simulink model "SimV6"  (R2024b)
settings: Solver=FixedStepAuto  StartTime=0.0  StopTime=5  RelTol=1e-3
model workspace (MAT data in the model file):
  Sig = Simulink.Signal
  Sig.Dimensions = -1
  Sig.DimensionsMode = 'auto'
  Sig.Complexity = 'auto'
  Sig.SampleTime = -1
  Sig.SamplingMode = 'auto'
  Sig.DataType = 'auto'
values from neighbouring files (symbols this model uses):
  CanaryCarrierFrequency = 20000.0    [ConfigData.sldd]
  CanaryDataRate = 100.0    [ConfigData.sldd]
  DataAmplitude = 10.0    [ConfigData.sldd]
  FmDecoderFrameSize = 128.0    [ConfigData.sldd]
  FmFrequencyDifferential = 400.0    [ConfigData.sldd]
  PreConvolveDownsample = 32.0    [ConfigData.sldd]
  SampleRate = 48000.0    [ConfigData.sldd]
  WalshCodeCache = 1.0 1.0 1.0 1.0 1.0 1.0 1.0 1.0 1.0 1.0 1.0 1.0 1.0 1.0 1.0 1.0 1.0 1.0 1.0 1.0 1.0 1.0 1.0 1.0 1.0 1.0 1.0 1.0 1.0 1.0 1.0 1.0 1.0 1.0 1.0 1.0 1.0 1.0 1.0 1.0 1.0 1.0 1.0 1.0 1.0 1.0 1.0 1.0 1.0 1.0 1.0 1.0 1.0 1.0 -1.0 -1.0 -1.0 -1.0 -1.0 -1.0 -1.0 -1.0 -1.0 -1.0 -1.0 -1.0 -1.0 -1.0 -1.0 -1.0 -1.0 -1.0 -1.0 -1.0 -1.0 -1.0 -1.0 -1.0 -1.0 -1.0 -1.0 -1.0 -1.0 -1.0 -1.0 -1.0 -1.0 -1.0 -1.0 -1.0 -1.0    [ConfigData.sldd]
  WalshCodeIndex = 3.0 9.0    [ConfigData.sldd]
libraries: dspstat3 x3, dspfdesign x3, audiosources x2, eeGeneralControl x2, commseqgen3 x2, commchan3 x1, dspsnks4 x1, simulink x1, dspsrcs4 x1, dspsigops x1
settings Model: DataDictionary=ConfigData.sldd  SimulationMode=accelerator  PauseTimes=4.5  PacingRate=0.007100  Creator=calum  LastModifiedBy=calum
settings SolverCC: AllowMultiTaskInputOutput=on  ConcurrentTasks=on  AutoInsertRateTranBlk=on
settings OptimizationCC: StateBitsets=on  DataBitsets=on  SimCompilerOptimization=on  AccelVerboseBuild=on  MultiThreadedLoops=on
settings DebuggingCC: IntegerOverflowMsg=none  IntegerSaturationMsg=none
settings HardwareCC: ProdBitPerLong=64  ProdLongLongMode=on  ProdHWDeviceType=Intel->x86-64 (Linux 64)
settings ModelReferenceCC: UpdateModelReferenceTargets=IfOutOfDate  EnableParallelModelReferenceBuilds=on  ParallelModelReferenceMATLABWorkerInit=Copy Base Workspace
settings SFSimCC: SimCtrlC=off  SimHardwareAcceleration=native
settings RTWCC: Description=Simulink Desktop Real-Time (ERT)  SystemTargetFile=sldrtert.tlc  TemplateMakefile=sldrtert.tmf  GenerateReport=on  Toolchain=GNU gcc/g++ | gmake (64-bit Linux)  BuildConfiguration=Specify  LaunchReport=on  TargetLang=C++  RTWCompilerOptimization=on  CheckMdlBeforeBuild=Warning
settings CodeAppCC: MaxIdLength=95  MATLABSourceComments=on
settings SimulinkDesktopRealTimeERTCC: TargetFcnLib=ansi_tfl_table_tmw.mat  TargetLibSuffix=_sldrt.a  TargetPreCompLibLocation=/home/calum/.local/matlab/2024b/toolbox/sldrt/lib/glnxa64  GenFloatMathFcnCalls=NOT IN USE  TargetLangStandard=C++11 (ISO)  CodeReplacementLibrary=None  UtilityFuncGeneration=Auto  MultiwordTypeDef=System defined  MultiwordLength=2048  DynamicStringBufferSize=256  GenerateFullHeader=on  InferredTypesCompatibility=off  GenerateSampleERTMain=off  GenerateTestInterfaces=off  ModelReferenceCompliant=on  ParMdlRefBuildCompliant=on  CompOptLevelCompliant=on  ConcurrentExecutionCompliant=off  IncludeMdlTerminateFcn=on  CombineOutputUpdateFcns=off  CombineSignalStateStructs=off  GroupInternalDataByFunction=off  SuppressErrorStatus=off  IncludeFileDelimiter=Auto  ERTCustomFileBanners=off  SupportAbsoluteTime=on  LogVarNameModifier=rt_  MatFileLogging=off  CodeInterfacePackaging=Nonreusable function  PurelyIntegerCode=off  SupportNonFinite=on  SupportComplex=on  SupportContinuousTime=on  SupportNonInlinedSFcns=on  RemoveDisableFunc=off  RemoveResetFunc=off  SupportVariableSizeSignals=on  ParenthesesLevel=Nominal  CastingMode=Nominal  MATLABClassNameForMDSCustomization=Simulink.SoftwareTarget.TargetSpecificTriggerConfigurationBase  ModelStepFunctionPrototypeControlCompliant=off  CPPClassGenCompliant=off  AutosarCompliant=off  MDXCompliant=off  GRTInterface=off  GenerateAllocFcn=off  UseToolchainInfoCompliant=off  GenerateSharedConstants=on  CoderGroups=[]  AccessMethods=[]  LookupTableObjectStructAxisOrder=1,2,3,4,...  LUTObjectStructOrderExplicitValues=Size,Breakpoints,Table  LUTObjectStructOrderEvenSpacing=Size,Breakpoints,Table  ArrayLayout=Column-major  UnsupportedSFcnMsg=error  ERTHeaderFileRootName=$R$E  ERTSourceFileRootName=$R$E  ERTDataFileRootName=$R_data  InstructionSetFMA=on  OptimizeReductions=on  LogToMDFFile=off  GenerateASAP2=off  DSAsUniqueAccess=off  ExtMode=on  ExtModeTransport=0  ExtModeStaticAlloc=off  ExtModeAutomaticAllocSize=on  ExtModeMaxTrigDuration=10  ExtModeStaticAllocSize=1000000  ExtModeTesting=off  ExtModeMexFile=sldrtext  ExtModeIntrfLevel=Level1  InlinedParameterPlacement=Hierarchical  TargetOS=BareBoardExample  MultiInstanceErrorCode=Error  RootIOFormat=Individual arguments  RTWCAPISignals=off  RTWCAPIParams=off  RTWCAPIStates=off  RTWCAPIRootIO=off  ERTSrcFileBannerTemplate=ert_code_template.cgt  ERTHdrFileBannerTemplate=ert_code_template.cgt  ERTDataSrcFileTemplate=ert_code_template.cgt  ERTDataHdrFileTemplate=ert_code_template.cgt  ERTCustomFileTemplate=example_file_process.tlc  EnableDataOwnership=off  SignalDisplayLevel=10  ParamTuneLevel=10  GlobalDataDefinition=Auto  DataDefinitionFile=global.c  GlobalDataReference=Auto  ERTFilePackagingFormat=Modular  RateTransitionBlockCode=Inline  DataReferenceFile=global.h  PreserveExpressionOrder=off  PreserveIfCondition=off  ConvertIfToSwitch=off  PreserveExternInFcnDecls=on  PreserveStaticInFcnDecls=on  SuppressUnreachableDefaultCases=off  EnableSignedLeftShifts=on  EnableSignedRightShifts=on  ImplementImageWithCVMat=off  IndentStyle=K&R  IndentSize=2  NewlineStyle=Default  MaxLineWidth=80  EnableUserReplacementTypes=off  MaxIdInt64=MAX_int64_T  MinIdInt64=MIN_int64_T  MaxIdUint64=MAX_uint64_T  MaxIdInt32=MAX_int32_T  MinIdInt32=MIN_int32_T  MaxIdUint32=MAX_uint32_T  MaxIdInt16=MAX_int16_T  MinIdInt16=MIN_int16_T  MaxIdUint16=MAX_uint16_T  MaxIdInt8=MAX_int8_T  MinIdInt8=MIN_int8_T  MaxIdUint8=MAX_uint8_T  BooleanTrueId=true  BooleanFalseId=false  MemSecPackage=--- None ---  MemSecDataConstants=Default  MemSecDataIO=Default  MemSecDataInternal=Default  MemSecDataParameters=Default  MemSecFuncInitTerm=Default  MemSecFuncExecute=Default  MemSecFuncSharedUtil=Default  GroupConstants=Default  GroupRootInputs=Default  GroupRootOutputs=Default  GroupInternal=Default  GroupParameters=Default  GroupDataTransfer=Default  GroupSharedLocalDataStores=Default  GroupInstanceSpecificParameters=Default  GroupModelData=Default  ArrayContainerType=C-style array  DynamicArrayContainerType=std::vector  CCListing=off  RebuildAll=off

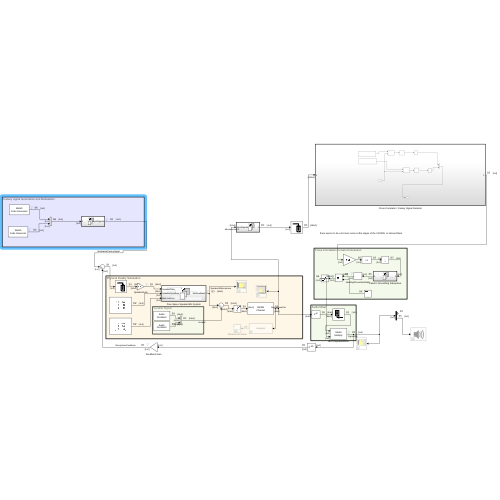
[thumbnail: Simulink's stored preview of the top-level diagram]
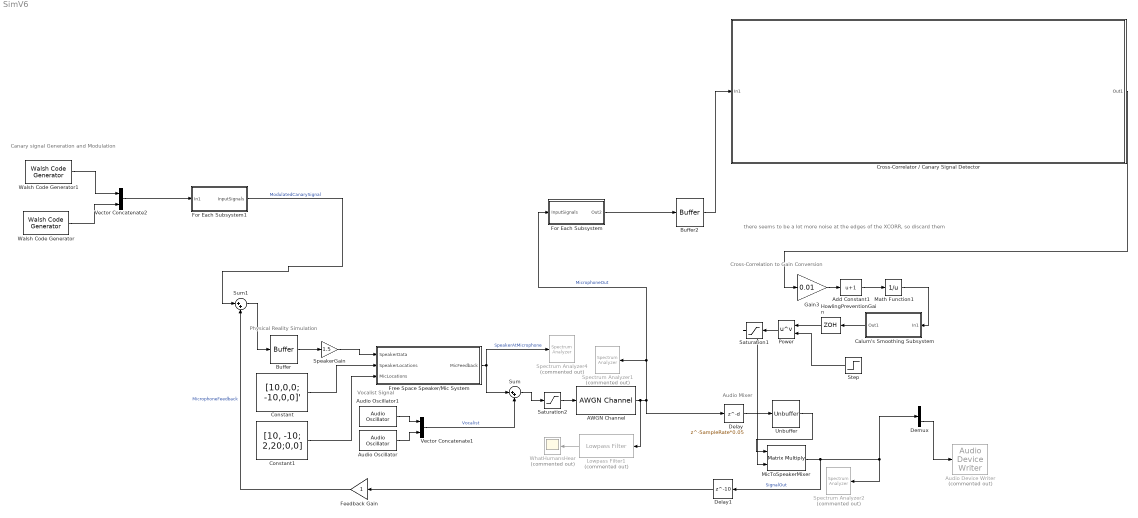
== system SimV6 ==
  note: Canary signal Generation and Modulation
  note: Audio Mixer
  note: Physical Reality Simulation
  note: Vocalist Signal
  note: Cross-Correlation to Gain Conversion
  note: there seems to be a lot more noise at the edges of the XCORR, so discard them
  AWGN Channel : commchan3/AWGN Channel  LegacyMode=off  NoiseMethod="Signal to noise ratio  (SNR)"  noiseMode="Signal to noise ratio  (SNR)"  EbNo=10  EsNo=10  SNR=60  BitsPerSymbol=1  SignalPower=1  SamplesPerSymbol=1  SymbolPeriod=1  VarianceSource=Parameter  Variance=1  RandomStream=Global stream  Seed=67  SimulateUsing=Code generation
  Add Constant1 : Bias  Bias=1  SaturateOnIntegerOverflow=off
  Audio Device Writer : dspsnks4/Audio Device Writer  Commented=on  Driver=ALSA  Device=Default  InheritSampleRate=on  SampleRate=44100  BitDepth=16-bit integer  BufferSize=4096  NumBuffers=10  DefaultOutputChannelMapping=on  OutputChannelMapping=1:2  OutputNumUnderrunSamples=off  DriverIdx=8  DeviceWarnFlag=''
  Audio Oscillator : audiosources/Audio Oscillator  FrequencyPort=off  Frequency=200  AmplitudePort=off  Amplitude=DataAmplitude  DCOffsetPort=off  DCOffset=0  PhaseOffset=0  WidthPort=off  Width=1  DutyCyclePort=off  DutyCycle=0.5  SampsPerFrame=64  Fs=SampleRate  OutputDataType=double  SimulateUsing=Code generation
      settings: SignalType=sine
  Audio Oscillator1 : audiosources/Audio Oscillator  FrequencyPort=off  Frequency=400  AmplitudePort=off  Amplitude=DataAmplitude  DCOffsetPort=off  DCOffset=0  PhaseOffset=0  WidthPort=off  Width=1  DutyCyclePort=off  DutyCycle=0.5  SampsPerFrame=64  Fs=SampleRate  OutputDataType=double  SimulateUsing=Code generation
      settings: SignalType=sine
  Buffer : Buffer  OutputFrames=off
  Buffer2 : Buffer  N=ceil(SampleRate/32/CanaryDataRate*32)+10  V=ceil(SampleRate/32/CanaryDataRate*32)+2  OutputFrames=off
  Calum's Smoothing Subsystem : Subsystem  TreatAsAtomicUnit=on
  Constant : Constant  Value="[10,0,0;  -10,0,0]'"
  Constant1 : Constant  Value=[10, -10; 2,20;0,0]
  "Cross-Correlator / Canary Signal Detector " : Subsystem  TreatAsAtomicUnit=on
  Delay : Delay  DelayLength=SampleRate*0.05  InitialCondition=0  InputProcessing=Columns as channels (frame based)  UseCircularBuffer=on
  Delay1 : Delay  DelayLength=10  InitialCondition=0
  Demux : Demux  Outputs=2
  Feedback Gain : Gain
  For Each Subsystem : Subsystem  TreatAsAtomicUnit=on
  For Each Subsystem1 : Subsystem  TreatAsAtomicUnit=on
  Free Space Speaker/Mic System : Subsystem  TreatAsAtomicUnit=on
  Gain3 : Gain  Gain=0.01
  HowlingPreventionGain : ZeroOrderHold  SampleTime=1/(CanaryDataRate)
  Lowpass Filter1 : dspfdesign/Lowpass Filter  Commented=on  FilterType=FIR  DesignForMinimumOrder=on  FilterOrder=50  PassbandFrequency=CanaryCarrierFrequency-8000  StopbandFrequency=CanaryCarrierFrequency-1000  PassbandRipple=0.1  StopbandAttenuation=80  SampleRateMode=Specify on dialog  SampleRate=SampleRate  SimulateUsing=Code generation  roundingMode=Floor  coeffsDataTypeStr=fixdt(1,16)
  Math Function1 : Math  Operator=reciprocal
  MicToSpeakerMixer : Product  Multiplication=Matrix(*)
  Power : Math  Operator=pow
  Saturation1 : Saturate  UpperLimit=1  LowerLimit=0
  Saturation2 : Saturate  UpperLimit=1000  LowerLimit=-1000
  SpeakerGain : Gain  Gain=1.5
  Spectrum Analyzer1 : SpectrumAnalyzer  Commented=on  WindowPosition=[1.000000,38.000000,1920.000000,1003.000000,]  ScopeFrameLocation=window  SampleRateSource=Property  SampleRate=SampleRate  PlotAsTwoSidedSpectrum=off  FrequencyScale=Log  FrequencySpan=Start and stop frequencies  StartFrequency=20  StopFrequency=20e3  YLimits=[-78.74086897,62.76889366]
  Spectrum Analyzer2 : SpectrumAnalyzer  Commented=on  WindowPosition=[1.000000,38.000000,1920.000000,1003.000000,]  ScopeFrameLocation=window  SampleRateSource=Property  SampleRate=SampleRate  PlotAsTwoSidedSpectrum=off  FrequencyScale=Log  FrequencySpan=Start and stop frequencies  StartFrequency=20  StopFrequency=20e3  YLimits=[-81.26361088,68.62221432]
  Spectrum Analyzer4 : SpectrumAnalyzer  Commented=on  WindowPosition=[1.000000,38.000000,1920.000000,1003.000000,]  ScopeFrameLocation=window  ViewType=Spectrum and spectrogram  SampleRateSource=Property  SampleRate=SampleRate  PlotAsTwoSidedSpectrum=off  FrequencyScale=Log  FrequencySpan=Start and stop frequencies  StartFrequency=20  StopFrequency=20e3  YLimits=[-136.03313301,69.13471038]  ColorLimits=[-136.03313301,69.13471038]
  Step : Step  Time=35  Before=5  After=0  SampleTime=1/(CanaryDataRate)
  Sum : Sum  Inputs=|++
  Sum1 : Sum  Inputs=|++
  Unbuffer : Unbuffer
  Vector Concatenate1 : Concatenate  Mode=Multidimensional array  ConcatenateDimension=2
  Vector Concatenate2 : Concatenate  Mode=Multidimensional array
  Walsh Code Generator : commseqgen3/Walsh Code Generator  Length=16  Index=WalshCodeIndex(2)  SampleTime=1/CanaryDataRate  SamplesPerFrame=1  OutputDataType=double  SimulateUsing=Code generation
  Walsh Code Generator1 : commseqgen3/Walsh Code Generator  Length=16  Index=WalshCodeIndex(1)  SampleTime=1/CanaryDataRate  SamplesPerFrame=1  OutputDataType=double  SimulateUsing=Code generation
  WhatHumansHear : Scope  Commented=on
  wires:
  Buffer/1 -> SpeakerGain/1
  Walsh Code Generator1/1 -> Vector Concatenate2/1
  AWGN Channel/1 -> Lowpass Filter1/1, For Each Subsystem/1(InputSignals), Spectrum Analyzer1/1, Delay/1  "MicrophoneOut"
  SpeakerGain/1 -> Free Space Speaker/Mic System/1(SpeakerData)
  Constant/1 -> Free Space Speaker/Mic System/2(SpeakerLocations)
  Constant1/1 -> Free Space Speaker/Mic System/3(MicLocations)
  Audio Oscillator1/1 -> Vector Concatenate1/1
  Audio Oscillator/1 -> Vector Concatenate1/2
  Add Constant1/1 -> Math Function1/1
  Gain3/1 -> Add Constant1/1
  Vector Concatenate1/1 -> Sum/2  "Vocalist"
  Free Space Speaker/Mic System/1(MicFeedback) -> Sum/1, Spectrum Analyzer4/1  "SpeakerAtMicrophone"
  Sum/1 -> Saturation2/1
  Math Function1/1 -> Calum's Smoothing Subsystem/1(In1)
  MicToSpeakerMixer/1 -> Demux/1, Spectrum Analyzer2/1, Delay1/1  "SignalOut"
  Calum's Smoothing Subsystem/1(Out1) -> HowlingPreventionGain/1
  Sum1/1 -> Buffer/1
  HowlingPreventionGain/1 -> Power/1
  Step/1 -> Power/2
  For Each Subsystem1/1(InputSignals) -> Sum1/1  "ModulatedCanarySignal"
  Power/1 -> Saturation1/1
  Saturation1/1 -> MicToSpeakerMixer/2
  Saturation2/1 -> AWGN Channel/1
  Feedback Gain/1 -> Sum1/2  "MicrophoneFeedback"
  Lowpass Filter1/1 -> WhatHumansHear/1
  Buffer2/1 -> "Cross-Correlator / Canary Signal Detector "/1(In1)
  "Cross-Correlator / Canary Signal Detector "/1(Out1) -> Gain3/1
  Walsh Code Generator/1 -> Vector Concatenate2/2
  Vector Concatenate2/1 -> For Each Subsystem1/1(In1)
  For Each Subsystem/1(Out2) -> Buffer2/1
  Demux/2 -> Audio Device Writer/1
  Unbuffer/1 -> MicToSpeakerMixer/1
  Delay1/1 -> Feedback Gain/1
  Delay/1 -> Unbuffer/1

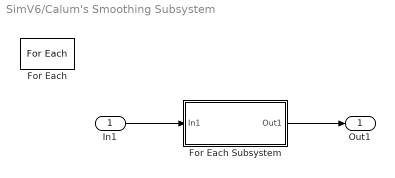
== system SimV6/Calum's Smoothing Subsystem ==
  In1 : Inport  Partition=on  PartitionDimension=1  PartitionWidth=1  PartitionOffset=0
  For Each : ForEach  DisableCoverage=on
  For Each Subsystem : Subsystem  TreatAsAtomicUnit=on
  Out1 : Outport  ConcatenationDimension=1
  wires:
  In1/1 -> For Each Subsystem/1(In1)
  For Each Subsystem/1(Out1) -> Out1/1

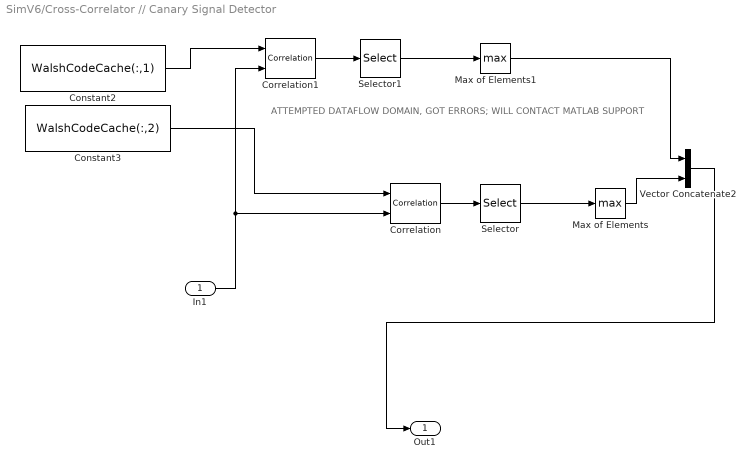
== system SimV6/Cross-Correlator // Canary Signal Detector  ==
  note: ATTEMPTED DATAFLOW DOMAIN, GOT ERRORS; WILL CONTACT MATLAB SUPPORT
  In1 : Inport
  Constant2 : Constant  Value=WalshCodeCache(:,1)  VectorParams1D=off
  Constant3 : Constant  Value=WalshCodeCache(:,2)  VectorParams1D=off
  Correlation : dspstat3/Correlation  domain=Time  roundingMode=Floor  overflowMode=off  outputDataTypeStr=Inherit: Same as accumulator  outputMin=[]  outputMax=[]  outputLastDataTypeStr=Inherit: Same as accumulator
  Correlation1 : dspstat3/Correlation  domain=Fastest  roundingMode=Floor  overflowMode=off  outputDataTypeStr=Inherit: Same as accumulator  outputMin=[]  outputMax=[]  outputLastDataTypeStr=Inherit: Same as accumulator
  Max of Elements : MinMax  Function=max  CollapseMode=Specified dimension
  Max of Elements1 : MinMax  Function=max  CollapseMode=Specified dimension
  Selector : Selector  NumberOfDimensions=2  InputPortWidth=3  IndexOptions=Index vector (dialog),Select all  Indices=[225 : 225+221],1  OutputSizes=1,1
  Selector1 : Selector  NumberOfDimensions=2  InputPortWidth=3  IndexOptions=Index vector (dialog),Select all  Indices=[225 : 225+221],1  OutputSizes=1,1
  Vector Concatenate2 : Concatenate  Mode=Multidimensional array
  Out1 : Outport
  wires:
  Constant2/1 -> Correlation1/1
  Selector/1 -> Max of Elements/1
  Constant3/1 -> Correlation/1
  Max of Elements1/1 -> Vector Concatenate2/1
  Max of Elements/1 -> Vector Concatenate2/2
  Correlation/1 -> Selector/1
  Correlation1/1 -> Selector1/1
  In1/1 -> Correlation/2, Correlation1/2
  Selector1/1 -> Max of Elements1/1
  Vector Concatenate2/1 -> Out1/1

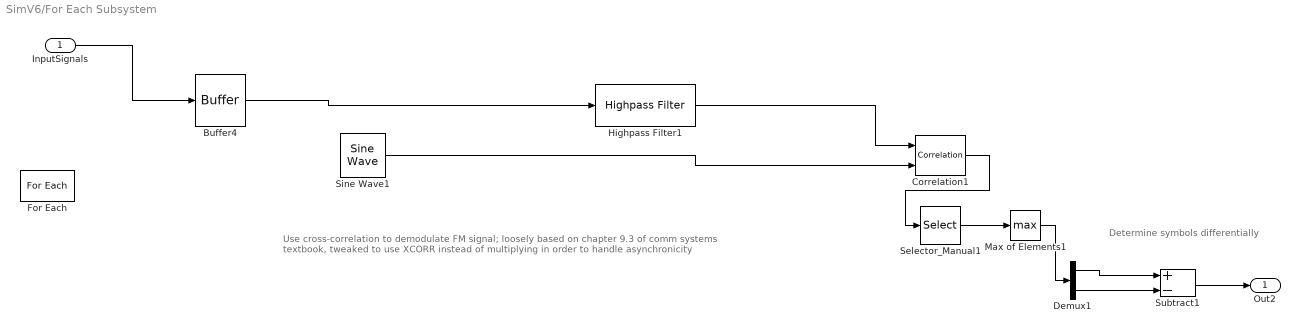
== system SimV6/For Each Subsystem ==
  note: Use cross-correlation to demodulate FM signal; loosely based on chapter 9.3 of comm systems textbook, tweaked to use XCORR instead of multiplying in order to handle asynchronicity
  note: Determine symbols differentially
  InputSignals : Inport  Partition=on  PartitionDimension=2  PartitionWidth=1  PartitionOffset=0
  Buffer4 : Buffer  N=FmDecoderFrameSize  V=FmDecoderFrameSize-PreConvolveDownsample  OutputFrames=off
  Correlation1 : dspstat3/Correlation  domain=Time  roundingMode=Floor  overflowMode=off  outputDataTypeStr=Inherit: Same as accumulator  outputMin=[]  outputMax=[]  outputLastDataTypeStr=Inherit: Same as accumulator
  Demux1 : Demux  Outputs=2
  For Each : ForEach  DisableCoverage=on
  Highpass Filter1 : dspfdesign/Highpass Filter  FilterType=FIR  DesignForMinimumOrder=on  FilterOrder=50  StopbandFrequency=CanaryCarrierFrequency-FmFrequencyDifferential*4  PassbandFrequency=CanaryCarrierFrequency-FmFrequencyDifferential  StopbandAttenuation=80  PassbandRipple=0.1  SampleRateMode=Specify on dialog  SampleRate=SampleRate  SimulateUsing=Code generation  roundingMode=Floor  coeffsDataTypeStr=fixdt(1,16)
  Max of Elements1 : MinMax  Function=max  CollapseMode=Specified dimension
  Selector_Manual1 : Selector  NumberOfDimensions=2  InputPortWidth=3  IndexOptions=Starting index (dialog),Select all  Indices=FmDecoderFrameSize/2,1  OutputSizes=FmDecoderFrameSize,1
  Sine Wave1 : dspsrcs4/Sine Wave  Amplitude=1  Frequency=[CanaryCarrierFrequency-FmFrequencyDifferential,CanaryCarrierFrequency+FmFrequencyDifferential]  Phase=0  SampleMode=Discrete  OutComplex=Real  CompMethod=Trigonometric fcn  TableSize=Speed  SampleTime=1/SampleRate  SamplesPerFrame=FmDecoderFrameSize  ResetState=Restart at time zero  OutputFrames=off  dataType=double  wordLen=16  udDataType=sfix(16)  fracBitsMode=Best precision  numFracBits=15  OutDataTypeStr=double  LastOutDataTypeStr=double
  Subtract1 : Sum  Inputs=+-
  Out2 : Outport  ConcatenationDimension=2
  wires:
  InputSignals/1 -> Buffer4/1
  Demux1/2 -> Subtract1/2
  Selector_Manual1/1 -> Max of Elements1/1
  Demux1/1 -> Subtract1/1
  Subtract1/1 -> Out2/1
  Max of Elements1/1 -> Demux1/1
  Highpass Filter1/1 -> Correlation1/1
  Sine Wave1/1 -> Correlation1/2
  Buffer4/1 -> Highpass Filter1/1
  Correlation1/1 -> Selector_Manual1/1

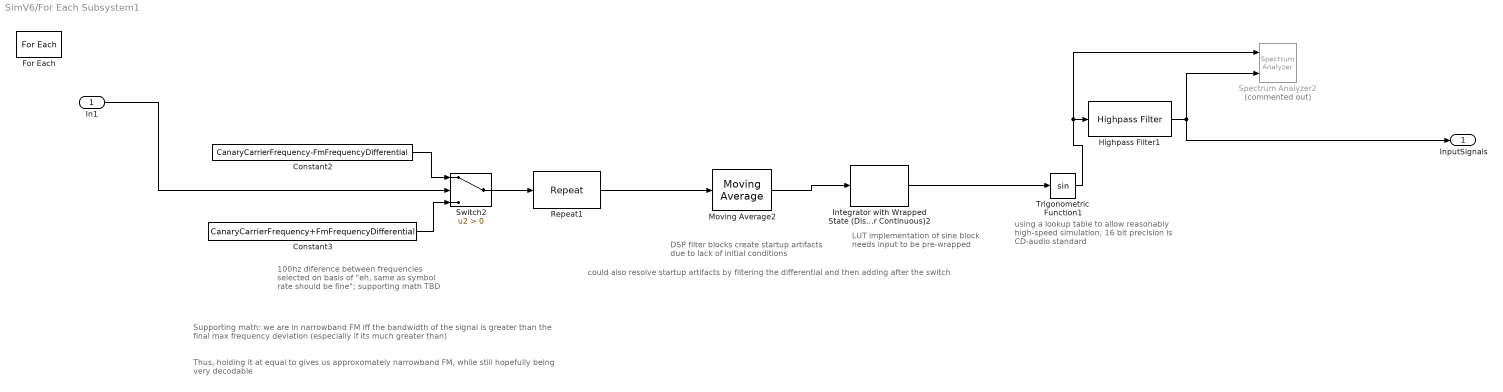
== system SimV6/For Each Subsystem1 ==
  note: could also resolve startup artifacts by filtering the differential and then adding after the switch
  note: Thus, holding it at equal to gives us approxomately narrowband FM, while still hopefully being very decodable
  note: Supporting math: we are in narrowband FM iff the bandwidth of the signal is greater than the final max frequency deviation (especially if its much greater than)
  note: 100hz diference between frequencies selected on basis of "eh, same as symbol rate should be fine"; supporting math TBD
  note: DSP filter blocks create startup artifacts
      | due to lack of initial conditions
  note: LUT implementation of sine block needs input to be pre-wrapped
  note: using a lookup table to allow reasonably high-speed simulation; 16 bit precision is CD-audio standard
  In1 : Inport  Partition=on  PartitionDimension=1  PartitionWidth=1  PartitionOffset=0
  Constant2 : Constant  Value=CanaryCarrierFrequency-FmFrequencyDifferential
  Constant3 : Constant  Value=CanaryCarrierFrequency+FmFrequencyDifferential
  For Each : ForEach  DisableCoverage=on
  Highpass Filter1 : dspfdesign/Highpass Filter  FilterType=FIR  DesignForMinimumOrder=on  FilterOrder=50  StopbandFrequency=CanaryCarrierFrequency-FmFrequencyDifferential*6  PassbandFrequency=CanaryCarrierFrequency-FmFrequencyDifferential  StopbandAttenuation=80  PassbandRipple=0.1  SampleRateMode=Specify on dialog  SampleRate=SampleRate  SimulateUsing=Code generation  roundingMode=Floor  coeffsDataTypeStr=fixdt(1,16)
  Integrator with Wrapped State (Discrete or Continuous)2 : eeGeneralControl/Integrator with Wrapped State (Discrete or Continuous)  LabelModeActiveChoice=Discrete  WrappedStateUpperValue=1  WrappedStateLowerValue=0  x0=0  Ts=-1
  Moving Average2 : eeGeneralControl/Moving Average  VariantControl=Variant1  LabelModeActiveChoice=Discrete  f=CanaryDataRate*4  x0=CanaryCarrierFrequency  BufferSize=8192  Ts=-1
  Repeat1 : dspsigops/Repeat  FactorSource=Dialog parameter  N=SampleRate/CanaryDataRate  Nmax=16  InputProcessing=Columns as channels (frame based)  RateOptions=Allow multirate processing  ic=CanaryCarrierFrequency  mode=Unused parameter value
  Spectrum Analyzer2 : SpectrumAnalyzer  Commented=on  NumInputPorts=2  WindowPosition=[1.000000,1.000000,1920.000000,1003.000000,]  Visible=on  ScopeFrameLocation=window  ViewType=Spectrum and spectrogram  SampleRate=44.1e3  FrequencyScale=Log  WindowInvariantSamplesPerUpdate=on  StartFrequency=20  StopFrequency=20e3  YLimits=[-118.30707698,33.34673002]  ColorLimits=[-118.30707698,33.34673002]  SelectedToolstripTab=spectrumAnalyzerToolstrip.spectrogramTab
  Switch2 : Switch  Criteria=u2 > Threshold  SaturateOnIntegerOverflow=off  InputSameDT=off
  Trigonometric Function1 : Trigonometry  ApproximationMethod=Lookup  AngleUnit=revolution  NumberOfDataPoints=(2^16)+1
  InputSignals : Outport  ConcatenationDimension=2
  wires:
  In1/1 -> Switch2/2
  Repeat1/1 -> Moving Average2/1
  Switch2/1 -> Repeat1/1
  Constant2/1 -> Switch2/1
  Constant3/1 -> Switch2/3
  Moving Average2/1 -> Integrator with Wrapped State (Discrete or Continuous)2/1
  Highpass Filter1/1 -> InputSignals/1, Spectrum Analyzer2/2
  Trigonometric Function1/1 -> Spectrum Analyzer2/1, Highpass Filter1/1
  Integrator with Wrapped State (Discrete or Continuous)2/1 -> Trigonometric Function1/1

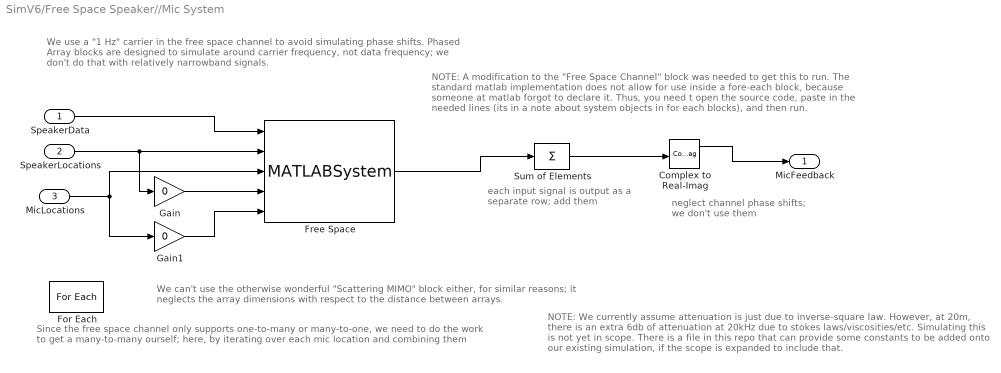
== system SimV6/Free Space Speaker//Mic System ==
  note: NOTE: We currently assume attenuation is just due to inverse-square law.
      | However, at 20m, there is an extra 6db of attenuation at 20kHz due to stokes laws/viscosities/etc.  Simulating this is not yet in scope.  There is a file in this repo that can provide some constants to be added onto our existing simulation, if the scope is expanded to include that.
  note: neglect channel phase
      | shifts; we don't use them
  note: each input signal is output as
      | a separate row; add them
  note: NOTE: A modification to the "Free Space Channel" block was needed to get
      | this to run.  The standard matlab implementation does not allow for use inside a fore-each block, because someone at matlab forgot to declare it.  Thus, you need t open the source code, paste in the needed lines (its in a note about system objects in for each blocks), and then run.
  note: Since the free space channel only supports one-to-many or many-to-one, we need to do the work to get a many-to-many ourself; here, by iterating over each mic location and combining them
  note: We can't use the otherwise wonderful "Scattering MIMO" block either, for similar reasons;
      | it neglects the array dimensions with respect to the distance between arrays.
  note: We use a "1 Hz" carrier in the free space channel to avoid simulating phase shifts.
      | Phased Array blocks are designed to simulate around carrier frequency, not data frequency; we don't do that
      | with relatively narrowband signals.
  SpeakerData : Inport
  SpeakerLocations : Inport  Port=2
  MicLocations : Inport  Port=3  Partition=on  PartitionDimension=2  PartitionWidth=1  PartitionOffset=0
  Complex to Real-Imag : ComplexToRealImag
  For Each : ForEach  DisableCoverage=on
  Free Space : MATLABSystem  System=FreeSpaceCalum  PropagationSpeed=SoundSpeed  OperatingFrequency=0.000001  TwoWayPropagation=off  SampleRateFromInputCheckbox=on  SampleRate=1e6  MaximumDistanceSource=Property  MaximumDistance=10e3  MaximumNumInputSamplesSource=Auto  MaximumNumInputSamples=100  SimulateUsing=Code generation
      settings: LibrarySourceBlock=phasedenvlib/Free Space
      mask Type: FreeSpaceCalum
      mask Display:
      | disp(['Free Space' char(10) 'Channel (Calum''s)']);
      | port_label('input',1,'X');
      | port_label('input',2,'Pos1');
      | port_label('input',3,'Pos2');
      | port_label('input',4,'Vel1');
      | port_label('input',5,'Vel2');
  Gain : Gain  Gain=0
  Gain1 : Gain  Gain=0
  Sum of Elements : Sum  Inputs=+  CollapseMode=Specified dimension  CollapseDim=2
  MicFeedback : Outport  ConcatenationDimension=2
  wires:
  SpeakerData/1 -> Free Space/1
  SpeakerLocations/1 -> Free Space/2, Gain/1
  Free Space/1 -> Sum of Elements/1
  Sum of Elements/1 -> Complex to Real-Imag/1
  Gain/1 -> Free Space/4
  Gain1/1 -> Free Space/5
  MicLocations/1 -> Gain1/1, Free Space/3
  Complex to Real-Imag/1 -> MicFeedback/1

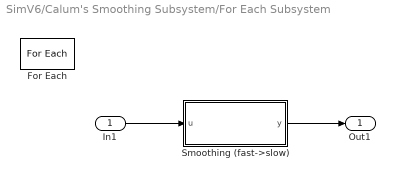
== system SimV6/Calum's Smoothing Subsystem/For Each Subsystem ==
  In1 : Inport  Partition=on  PartitionDimension=2  PartitionWidth=1  PartitionOffset=0
  For Each : ForEach  DisableCoverage=on
  Smoothing (fast->slow) : Subsystem  mask(Smoothing (fast->slow)){nSmooth=floor(SampleRate/CanaryDataRate/PreConvolveDownsample), h1=-1, smoothing0=1}
      mask prompts: nSmooth "physmod:simscape:couplers:SimscapeNetworkCouplersLib:NumberOfSamplesOverWhichToSmooth_MP"; h1 "physmod:simscape:couplers:SimscapeNetworkCouplersLib:PortUDiscreteSampleTimes_MP"; smoothing0 "physmod:simscape:couplers:SimscapeNetworkCouplersLib:InitialOutput_MP"
      mask help: physmod:simscape:couplers:SimscapeNetworkCouplersLib:Smoothingfastslow_MD
      mask Help: web([docroot '/simscape/ref/smoothingfastslow.html'])
      mask DialogControl nSmooth Prompt: Number of samples over which to smooth
      mask DialogControl h1 Prompt: Port u discrete sample time (s)
      mask DialogControl smoothing0 Prompt: Initial output
  Out1 : Outport  ConcatenationDimension=2
  wires:
  In1/1 -> Smoothing (fast->slow)/1(u)
  Smoothing (fast->slow)/1(y) -> Out1/1

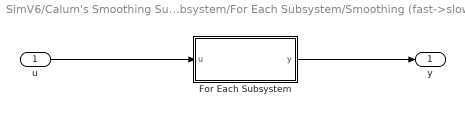
== system SimV6/Calum's Smoothing Subsystem/For Each Subsystem/Smoothing (fast->slow) ==
  u : Inport
  For Each Subsystem : Subsystem  TreatAsAtomicUnit=on
  y : Outport
  wires:
  For Each Subsystem/1(y) -> y/1
  u/1 -> For Each Subsystem/1(u)

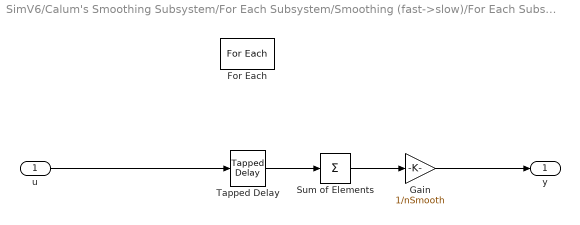
== system SimV6/Calum's Smoothing Subsystem/For Each Subsystem/Smoothing (fast->slow)/For Each Subsystem ==
  u : Inport  Partition=on  PartitionDimension=1  PartitionWidth=1  PartitionOffset=0
  For Each : ForEach  DisableCoverage=on
  Gain : Gain  Gain=1/nSmooth
  Sum of Elements : Sum  Inputs=+
  Tapped Delay : simulink/Discrete/Tapped Delay  vinit=mean(smoothing0)  samptime=h1  NumDelays=nSmooth  DelayOrder=Oldest  includeCurrent=off
  y : Outport  ConcatenationDimension=1
  wires:
  u/1 -> Tapped Delay/1
  Sum of Elements/1 -> Gain/1
  Tapped Delay/1 -> Sum of Elements/1
  Gain/1 -> y/1
